simulink model "CCCV"  (R2023a)
settings: Solver=VariableStepAuto  StartTime=0.0  StopTime=80  RelTol=1e-3
undefined symbols (not defined in the file): Ion, Lithium
libraries: spsMosfetLib x2, spsBatteryLib x1, spsControlledCurrentSourceLib x1, spsDCVoltageSourceLib x1, spsDiodeLib x1, spsSeriesRLCBranchLib x1, spspowerguiLib x1
settings Model: Creator=Siddesh  LastModifiedBy=Siddesh

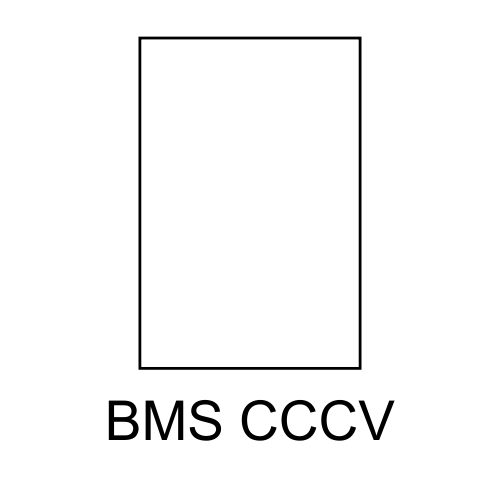
[thumbnail: Simulink's stored preview of the top-level diagram]
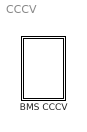
== system CCCV ==
  BMS CCCV : Subsystem

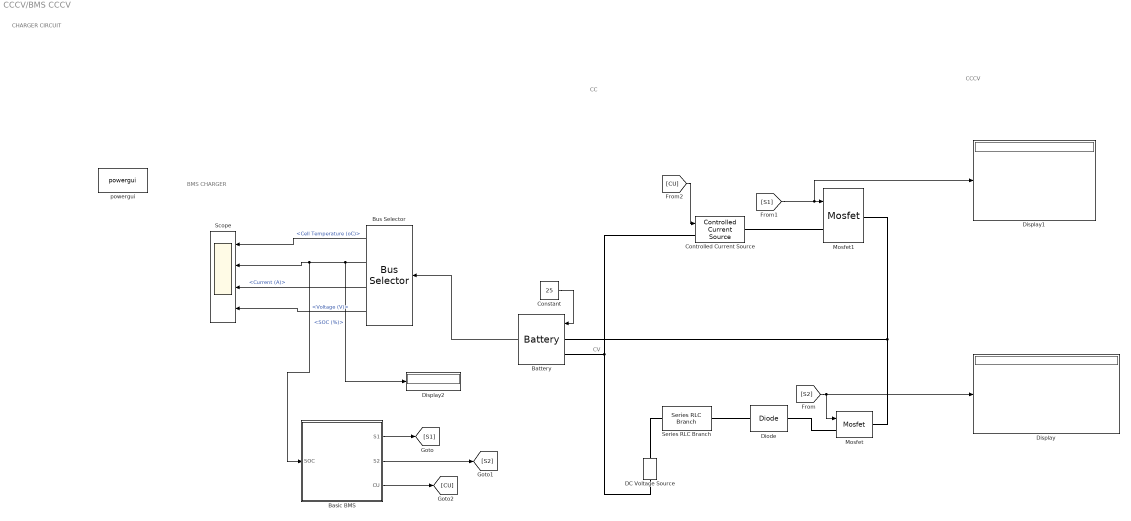
== system CCCV/BMS CCCV ==
  note: CHARGER CIRCUIT
  note: CCCV
  note: BMS CHARGER
  note: CV
  note: CC
  "Basic BMS " : MATLAB Function  TreatAsAtomicUnit=on
  Battery : spsBatteryLib/Battery  BatType=Lithium-Ion  ShowTempParam=on  ThermalPreset="3.3V  2.3Ah  (LiFePO4)"  ShowAgeParam=off  NomV=3.3  NomQ=2.3  SOC=79  Batt_Tr=30  PresetModel=off  MaxQ=2.3  MinV=2.475  FullV=3.748  Dis_rate=2.3  R=0.014  Normal_OP=2.25  expZone="[3.4788       0.113]"  current=[6.5 13 32.5]  Units=Time  Tci=20  NomT=25  T2=0  MaxQ2=2.208  FullV2=3.45  Normal_OP2=2.85  expZone2="[3.22       0.015]"  Rca=0.6  ti=1000  Dp=0  Neq0=0  Tsim=1e6  Ta1=25  Qeol=5.4*0.9  Reol=0.013333*1.2  Char_age=[2.3478, 3]  Dis_age=[2.3478, 10]  N1=1500  N2=10500  N3=1000  N4=1400  Ta2=45  N5=950
  Bus Selector : BusSelector  OutputSignals=Cell Temperature (oC),SOC (%),Current (A),Voltage (V)
  Constant : Constant  Value=25
  Controlled Current Source : spsControlledCurrentSourceLib/Controlled Current Source  Initialize=on  Source_Type=AC  Amplitude=0  Phase=0  Frequency=0  Measurements=None
  DC Voltage Source : spsDCVoltageSourceLib/DC Voltage Source  Amplitude=24  Measurements=None
  Diode : spsDiodeLib/Diode  Ron=0.001  Lon=0  Vf=0.8  IC=0  UseSnubber=0  Rs=500  Cs=250e-9  Measurements=off
  Display : Display
  Display1 : Display
  Display2 : Display
  Mosfet : spsMosfetLib/Mosfet  Ron=0.1  Lon=0  Rd=0.01  Vfd=0  IC=0  Rs=1e5  Cs=inf  Measurements=off
  Mosfet1 : spsMosfetLib/Mosfet  Ron=0.1  Lon=0  Rd=0.01  Vfd=0  IC=0  Rs=1e5  Cs=inf  Measurements=off
  Scope : Scope  NumInputPorts=4
  Series RLC Branch : spsSeriesRLCBranchLib/Series RLC Branch  LConnTagsString=__new0  RConnTagsString=__new0  BranchType=R  Resistance=1  Inductance=1e-3  SetiL0=off  InitialCurrent=0  Capacitance=1e-6  Setx0=off  InitialVoltage=0  Measurements=None
  powergui : spspowerguiLib/powergui  Priority=1  SimulationMode=Discrete  SampleTime=50e-6  frequency=60  Iterations=50  frequencyindice=0  Pbase=100e6  ErrMax=1e-4  UnitsV=kV  UnitsW=MW  buscounter=0  FunctionMessages=off  echomessages=off  EnableUseOfTLC=off  CurrentSourceSwitches=off  DisableSnubberDevices=off  DisableRonSwitches=off  DisableVfSwitches=off  DisplayEquations=off  AutomaticDiscreteSolvers=off  SolverType=Tustin/Backward Euler (TBE)  Interpol=off  ExternalGateDelay=off  methode=off  Ts=100  x0status=blocks  SPID=on  SwTol=0  HookPort=off  NonlinearTolerance=1e-4  nMaxIteration=100  ContinueOnMaxIteration=off  RestoreLinks=warning  ResistiveCurrentMeasurement=off  Frange=[0:2:500]  Ylog=off  Xlog=on  ShowGrid=off  save=off  variable=ZData  structure=0  ZoomFFT=off  StartTime=0.0  cycles=1  DisplayStyle=1  fundamental=60  FreqAxis=off  MaxFrequency=1000  frequencyindicesteady=1  RmsSteady=1  display=off
  wires:
  [CU] -> Controlled Current Source/1
  [S1] -> Display1/1, Mosfet1/1
  Bus Selector/2 -> Display2/1, "Basic BMS "/1(SOC), Scope/2  "<SOC (%)>"
  "Basic BMS "/1(S1) -> [S1]
  "Basic BMS "/3(CU) -> [CU]
  Battery/1 -> Bus Selector/1
  [S2] -> Mosfet/1, Display/1
  "Basic BMS "/2(S2) -> [S2]
  Constant/1 -> Battery/1
  Bus Selector/1 -> Scope/1  "<Cell Temperature (oC)>"
  Bus Selector/4 -> Scope/4  "<Voltage (V)>"
  Bus Selector/3 -> Scope/3  "<Current (A)>"
  connections:
  Diode/RConn1 -- Mosfet/LConn1
  Battery/LConn2 -- Controlled Current Source/LConn1 -- DC Voltage Source/LConn1
  Controlled Current Source/RConn1 -- Mosfet1/LConn1
  Series RLC Branch/LConn1 -- DC Voltage Source/RConn1
  Diode/LConn1 -- Series RLC Branch/RConn1
  Mosfet/RConn1 -- Mosfet1/RConn1 -- Battery/LConn1

== matlab function CCCV/BMS CCCV/Basic BMS  ==
  data: SOC input; S1 output; S2 output; CU output
function [S1, S2, CU] = fcn(SOC)

CU = 0;
if ((SOC == 0) || (SOC <= 50))
    S1 = 1;
    CU = 2;
    S2 = 0;    
elseif ((SOC >50) && (SOC <=80))
    S1 = 1;
    S2 = 0;
    CU = 4;
elseif ((SOC > 80) && (SOC < 90))
    S1 = 0;
    S2 = 1;
    CU = 2;
else 
    S1 = 0;
    S2 = 0;
end
